simulink model "ISReferenceApplication"  (R2018a)
settings: Solver=FixedStepAuto  StartTime=0  StopTime=Tend  FixedStep=0.001  RelTol=5e-3
model workspace (MAT data in the model file):
  A_mu = 10
  B_reff = 8.386
  Cz = 7766.25
  DCT_Param : struct (value not decoded)
  D_reff = 0.25826
  Downshift_Speeds = [9.5625 12.9375 16.3125 19.6875 23.0625 26.4375 29.8125 33.1875 36.5625 39.9375 43.3125 46.6875 ... (28 elements, 4x7)]
  Pedal_Positions = [0.1 0.4 0.5 0.9]
  SUS : struct (value not decoded)
  Upshift_Speeds = [12.9375 16.3125 19.6875 33 26.4375 29.8125 33.1875 52.5 39.9375 43.3125 46.6875 77.25 ... (28 elements, 4x7)]
  VEH : struct (value not decoded)
  V_o = 16.7
  V_xlow = 1
  WH : struct (value not decoded)
  a = 1.4
  alpha_max = 1.5
  alpha_min = -1.5
  b = 1.8
  c_zo = 209651
  epsilon = 0.1
  h = 0.134
  path : struct (value not decoded)
  pio = 220000
  q_Fcx = 0
  q_Fz2 = 15.4
  q_Fzy = 0
  q_reo = 0.9974
  q_sx1 = -0.007764
  q_sx10 = 0.2824
  q_sx11 = 5.349
  q_sx12 = 0
  q_sx13 = 0
  q_sx14 = 0
  q_sx2 = 1.1915
  q_sx3 = 0.013948
  q_sx4 = 4.912
  q_sx5 = 1.02
  q_sx6 = 22.83
  q_sx7 = 0.7104
  q_sx8 = -0.023393
  q_sx9 = 0.6581
  q_sy1 = 0.00702
  q_sy2 = 0
  q_sy3 = 0.001515
  q_sy4 = 8.514e-05
  q_sy5 = 0
  q_sy6 = 0
  q_sy7 = 0.9008
  q_sy8 = -0.4089
  q_v1 = 0.0007742
  q_v2 = 0.04667
  r_Bx1 = 12.531
  r_Bx2 = 9.532
  r_Bx3 = 0
  r_By1 = 10.615
  r_By2 = 7.705
  r_By3 = 3.433e-06
  r_By4 = 0
  r_Cx1 = 1.019
  r_Cy1 = 1.0585
  r_Ex1 = -0.4487
  r_Ex2 = -0.4726
  r_Ey1 = 0.3132
  r_Ey2 = 7.63e-06
  r_Hx1 = 0.0002374
  r_Hy1 = 0.011646
  r_Hy2 = 7.63e-06
  r_Vy1 = 0.05654
  r_Vy2 = 7.63e-06
  r_Vy3 = 0
  r_Vy4 = 99.9
  r_Vy5 = 2
  r_Vy6 = 15.814
  r_o = 0.3135
  vehWidth = 2
  w = 1
undefined symbols (not defined in the file): Cok_1, Cok_2, Cok_3, Cok_4, Cok_5, Cok_6, Cok_7, Cok_8, Cok_9, Cout_1, Cout_2, Cout_3, Cout_4, Cout_5, Cout_6, Cout_7, Cout_8, Cout_9, Dout_1, Dout_2, Dout_3, Dout_4, Dout_5, Dout_6, Dout_7, Dout_8, Dout_9, F_1, F_2, F_3, F_4, F_5, F_6, F_7, F_8, F_9, Gd_1, Gd_2, Gd_3, Gd_4, Gd_5, Gd_6, Gd_7, Gd_8, Gd_9, Gok_1, Gok_2, Gok_3, Gok_4, Gok_5, Gok_6, Gok_7, Gok_8, Gok_9, Hd_1, Hd_2, Hd_3, Hd_4, Hd_5, Hd_6 ... (+64)
(part 2 of 3)

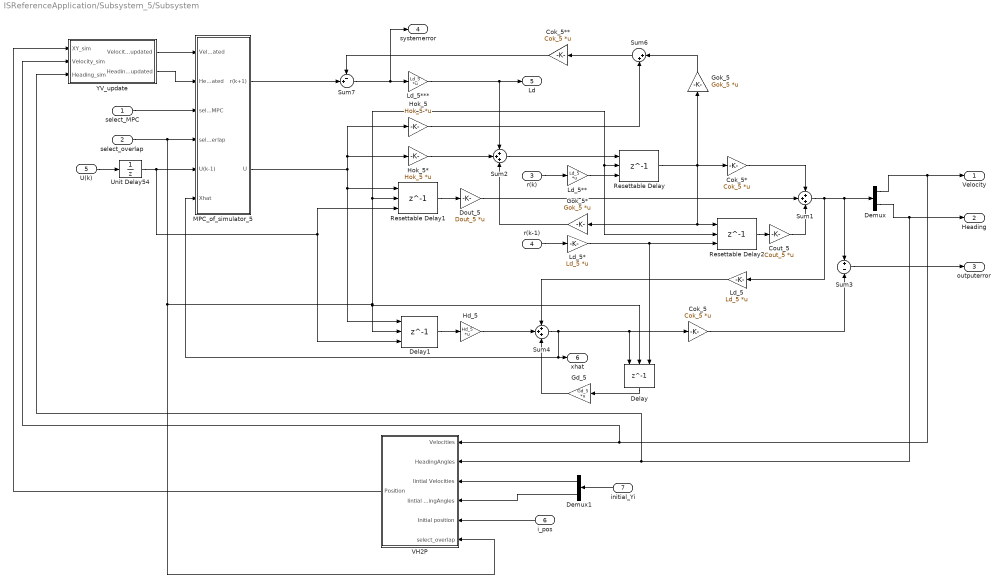
== system ISReferenceApplication/Subsystem_5/Subsystem ==
  select_MPC : Inport
  select_overlap : Inport  Port=2
  r(k) : Inport  Port=3
  r(k-1) : Inport  Port=4
  U(k) : Inport  Port=5
  i_pos : Inport  Port=6
  initial_Yi : Inport  Port=7
  Cok_5 : Gain  Gain=Cok_5  Multiplication=Matrix(K*u) (u vector)
  Cok_5* : Gain  Gain=Cok_5  Multiplication=Matrix(K*u) (u vector)
  Cok_5** : Gain  Gain=Cok_5  Multiplication=Matrix(K*u) (u vector)
  Cout_5 : Gain  Gain=Cout_5  Multiplication=Matrix(K*u) (u vector)
  Delay : Delay  DelayLength=1  InitialConditionSource=Input port  InitialCondition=0  ExternalReset=Rising  SampleTime=Ts
      settings: InputPortMap=u0,r5,p4
  Delay1 : Delay  DelayLength=1  InitialConditionSource=Input port  InitialCondition=0  ExternalReset=Rising  SampleTime=Ts
      settings: InputPortMap=u0,r5,p4
  Demux : Demux  Outputs=2
  Demux1 : Demux  Outputs=2
  Dout_5 : Gain  Gain=Dout_5  Multiplication=Matrix(K*u) (u vector)
  Gd_5 : Gain  Gain=Gd_5  Multiplication=Matrix(K*u) (u vector)
  Gok_5 : Gain  Gain=Gok_5  Multiplication=Matrix(K*u) (u vector)
  Gok_5* : Gain  Gain=Gok_5  Multiplication=Matrix(K*u) (u vector)
  Hd_5 : Gain  Gain=Hd_5  Multiplication=Matrix(K*u) (u vector)
  Hok_5 : Gain  Gain=Hok_5  Multiplication=Matrix(K*u) (u vector)
  Hok_5* : Gain  Gain=Hok_5  Multiplication=Matrix(K*u) (u vector)
  Ld_5 : Gain  Gain=Ld_5  Multiplication=Matrix(K*u) (u vector)
  Ld_5* : Gain  Gain=Ld_5  Multiplication=Matrix(K*u) (u vector)
  "Ld_5** " : Gain  Gain=Ld_5  Multiplication=Matrix(K*u) (u vector)
  Ld_5*** : Gain  Gain=Ld_5  Multiplication=Matrix(K*u) (u vector)
  MPC_of_simulator_5 : Subsystem
  Resettable Delay : Delay  DelayLength=1  InitialConditionSource=Input port  ExternalReset=Rising  SampleTime=Ts
      settings: InputPortMap=u0,r5,p4
  Resettable Delay1 : Delay  DelayLength=1  InitialConditionSource=Input port  ExternalReset=Rising  SampleTime=Ts
      settings: InputPortMap=u0,r5,p4
  Resettable Delay2 : Delay  DelayLength=1  InitialConditionSource=Input port  ExternalReset=Rising  SampleTime=Ts
      settings: InputPortMap=u0,r5,p4
  Sum1 : Sum  Inputs=+++
  Sum2 : Sum  Inputs=+++
  Sum3 : Sum  Inputs=+-
  Sum4 : Sum  Inputs=+++
  Sum6 : Sum  Inputs=|++
  Sum7 : Sum  Inputs=-+|
  Unit Delay54 : UnitDelay  SampleTime=Ts
  VH2P : Subsystem
  YV_update : Subsystem  TreatAsAtomicUnit=on
  Velocity : Outport
  Heading : Outport  Port=2
  outputerror : Outport  Port=3
  systemerror : Outport  Port=4
  Ld : Outport  Port=5
  xhat : Outport  Port=6
  wires:
  U(k)/1 -> Unit Delay54/1
  Cok_5*/1 -> Sum1/1
  Resettable Delay/1 -> Gok_5*/1, Resettable Delay2/1, Cok_5*/1, Gok_5/1
  Dout_5/1 -> Sum1/2
  Sum7/1 -> systemerror/1, Ld_5***/1
  r(k)/1 -> "Ld_5** "/1
  Gok_5*/1 -> Sum2/3
  Cout_5/1 -> Sum1/3
  Sum2/1 -> Resettable Delay/1
  "Ld_5** "/1 -> Resettable Delay/3
  Resettable Delay2/1 -> Cout_5/1
  r(k-1)/1 -> Ld_5*/1
  Hok_5/1 -> Sum6/2
  Gok_5/1 -> Sum6/1
  Resettable Delay1/1 -> Dout_5/1
  Sum6/1 -> Cok_5**/1
  Cok_5**/1 -> Sum7/1
  Hok_5*/1 -> Sum2/2
  Ld_5*/1 -> Resettable Delay2/3, Delay/3
  MPC_of_simulator_5/2(U) -> Hok_5/1, Hok_5*/1, Delay1/1, Resettable Delay1/1
  MPC_of_simulator_5/1(r(k+1)) -> Sum7/2
  Sum4/1 -> Cok_5/1, Delay/1, MPC_of_simulator_5/6(Xhat), xhat/1
  Gd_5/1 -> Sum4/3
  Delay/1 -> Gd_5/1
  Delay1/1 -> Hd_5/1
  Sum1/1 -> Ld_5/1, Sum3/1, Demux/1
  Cok_5/1 -> Sum3/2
  Hd_5/1 -> Sum4/2
  Ld_5***/1 -> Ld/1, Sum2/1
  Sum3/1 -> outputerror/1
  YV_update/1(Velocity_updated) -> MPC_of_simulator_5/1(Velocity_updated)
  YV_update/2(Heading_updated) -> MPC_of_simulator_5/2(Heading_updated)
  select_MPC/1 -> MPC_of_simulator_5/3(select_MPC)
  Demux/2 -> YV_update/3(Heading_sim), VH2P/2(HeadingAngles), Heading/1
  Demux/1 -> YV_update/2(Velocity_sim), VH2P/1(Velocities), Velocity/1
  VH2P/1(Position) -> YV_update/1(XY_sim)
  select_overlap/1 -> Resettable Delay2/2, Resettable Delay/2, Resettable Delay1/2, Delay/2, Delay1/2, VH2P/6(select_overlap), MPC_of_simulator_5/4(select_overlap)
  Unit Delay54/1 -> Resettable Delay1/3, Delay1/3, MPC_of_simulator_5/5(U(k-1))
  initial_Yi/1 -> Demux1/1
  Ld_5/1 -> Sum4/1
  i_pos/1 -> VH2P/5(Initial position)
  Demux1/1 -> VH2P/3(Iintial Velocities)
  Demux1/2 -> VH2P/4(Iintial HeadingAngles)

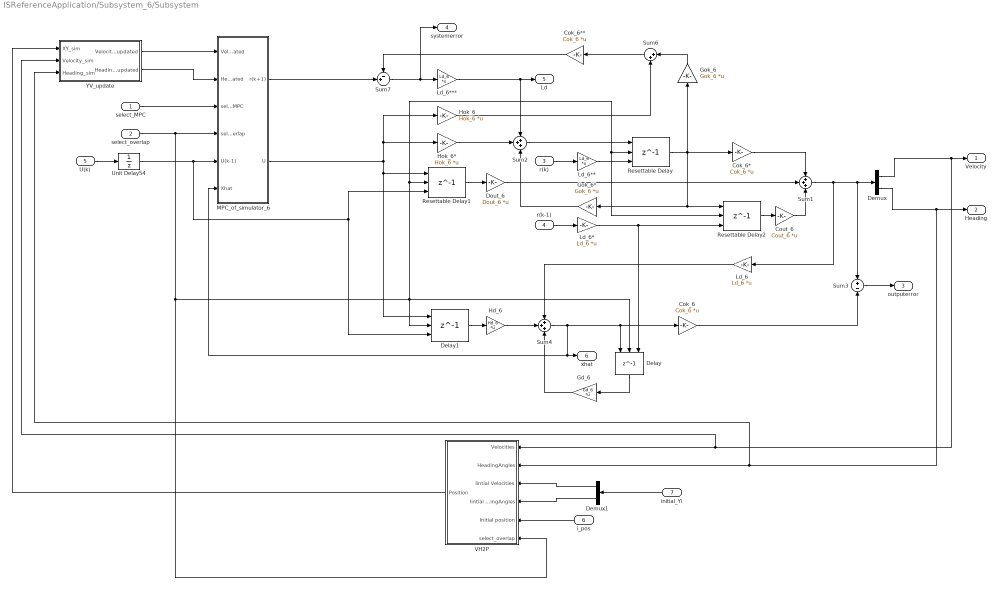
== system ISReferenceApplication/Subsystem_6/Subsystem ==
  select_MPC : Inport
  select_overlap : Inport  Port=2
  r(k) : Inport  Port=3
  r(k-1) : Inport  Port=4
  U(k) : Inport  Port=5
  i_pos : Inport  Port=6
  initial_Yi : Inport  Port=7
  Cok_6 : Gain  Gain=Cok_6  Multiplication=Matrix(K*u) (u vector)
  Cok_6* : Gain  Gain=Cok_6  Multiplication=Matrix(K*u) (u vector)
  Cok_6** : Gain  Gain=Cok_6  Multiplication=Matrix(K*u) (u vector)
  Cout_6 : Gain  Gain=Cout_6  Multiplication=Matrix(K*u) (u vector)
  Delay : Delay  DelayLength=1  InitialConditionSource=Input port  InitialCondition=0  ExternalReset=Rising  SampleTime=Ts
      settings: InputPortMap=u0,r5,p4
  Delay1 : Delay  DelayLength=1  InitialConditionSource=Input port  InitialCondition=0  ExternalReset=Rising  SampleTime=Ts
      settings: InputPortMap=u0,r5,p4
  Demux : Demux  Outputs=2
  Demux1 : Demux  Outputs=2
  Dout_6 : Gain  Gain=Dout_6  Multiplication=Matrix(K*u) (u vector)
  Gd_6 : Gain  Gain=Gd_6  Multiplication=Matrix(K*u) (u vector)
  Gok_6 : Gain  Gain=Gok_6  Multiplication=Matrix(K*u) (u vector)
  Gok_6* : Gain  Gain=Gok_6  Multiplication=Matrix(K*u) (u vector)
  Hd_6 : Gain  Gain=Hd_6  Multiplication=Matrix(K*u) (u vector)
  Hok_6 : Gain  Gain=Hok_6  Multiplication=Matrix(K*u) (u vector)
  Hok_6* : Gain  Gain=Hok_6  Multiplication=Matrix(K*u) (u vector)
  Ld_6 : Gain  Gain=Ld_6  Multiplication=Matrix(K*u) (u vector)
  Ld_6* : Gain  Gain=Ld_6  Multiplication=Matrix(K*u) (u vector)
  "Ld_6** " : Gain  Gain=Ld_6  Multiplication=Matrix(K*u) (u vector)
  Ld_6*** : Gain  Gain=Ld_6  Multiplication=Matrix(K*u) (u vector)
  MPC_of_simulator_6 : Subsystem
  Resettable Delay : Delay  DelayLength=1  InitialConditionSource=Input port  ExternalReset=Rising  SampleTime=Ts
      settings: InputPortMap=u0,r5,p4
  Resettable Delay1 : Delay  DelayLength=1  InitialConditionSource=Input port  ExternalReset=Rising  SampleTime=Ts
      settings: InputPortMap=u0,r5,p4
  Resettable Delay2 : Delay  DelayLength=1  InitialConditionSource=Input port  ExternalReset=Rising  SampleTime=Ts
      settings: InputPortMap=u0,r5,p4
  Sum1 : Sum  Inputs=+++
  Sum2 : Sum  Inputs=+++
  Sum3 : Sum  Inputs=+-
  Sum4 : Sum  Inputs=+++
  Sum6 : Sum  Inputs=|++
  Sum7 : Sum  Inputs=-+|
  Unit Delay54 : UnitDelay  SampleTime=Ts
  VH2P : Subsystem
  YV_update : Subsystem  TreatAsAtomicUnit=on
  Velocity : Outport
  Heading : Outport  Port=2
  outputerror : Outport  Port=3
  systemerror : Outport  Port=4
  Ld : Outport  Port=5
  xhat : Outport  Port=6
  wires:
  Sum2/1 -> Resettable Delay/1
  Sum6/1 -> Cok_6**/1
  Resettable Delay/1 -> Cok_6*/1, Resettable Delay2/1, Gok_6*/1, Gok_6/1
  Resettable Delay1/1 -> Dout_6/1
  Dout_6/1 -> Sum1/2
  Hok_6/1 -> Sum6/2
  MPC_of_simulator_6/2(U) -> Hok_6/1, Hok_6*/1, Delay1/1, Resettable Delay1/1
  r(k)/1 -> "Ld_6** "/1
  Sum1/1 -> Ld_6/1, Sum3/1, Demux/1
  Ld_6*/1 -> Resettable Delay2/3, Delay/3
  Hok_6*/1 -> Sum2/2
  Sum7/1 -> systemerror/1, Ld_6***/1
  Cok_6**/1 -> Sum7/1
  Cout_6/1 -> Sum1/3
  r(k-1)/1 -> Ld_6*/1
  Resettable Delay2/1 -> Cout_6/1
  "Ld_6** "/1 -> Resettable Delay/3
  Gok_6/1 -> Sum6/1
  Gok_6*/1 -> Sum2/3
  U(k)/1 -> Unit Delay54/1
  Ld_6***/1 -> Ld/1, Sum2/1
  Cok_6*/1 -> Sum1/1
  MPC_of_simulator_6/1(r(k+1)) -> Sum7/2
  Hd_6/1 -> Sum4/2
  Gd_6/1 -> Sum4/3
  Cok_6/1 -> Sum3/2
  Delay/1 -> Gd_6/1
  Delay1/1 -> Hd_6/1
  Sum4/1 -> Cok_6/1, Delay/1, MPC_of_simulator_6/6(Xhat), xhat/1
  Sum3/1 -> outputerror/1
  select_MPC/1 -> MPC_of_simulator_6/3(select_MPC)
  Demux/1 -> YV_update/2(Velocity_sim), VH2P/1(Velocities), Velocity/1
  VH2P/1(Position) -> YV_update/1(XY_sim)
  Demux/2 -> VH2P/2(HeadingAngles), YV_update/3(Heading_sim), Heading/1
  select_overlap/1 -> VH2P/6(select_overlap), Resettable Delay2/2, Resettable Delay/2, Resettable Delay1/2, Delay/2, Delay1/2, MPC_of_simulator_6/4(select_overlap)
  YV_update/1(Velocity_updated) -> MPC_of_simulator_6/1(Velocity_updated)
  YV_update/2(Heading_updated) -> MPC_of_simulator_6/2(Heading_updated)
  Unit Delay54/1 -> Resettable Delay1/3, Delay1/3, MPC_of_simulator_6/5(U(k-1))
  initial_Yi/1 -> Demux1/1
  Ld_6/1 -> Sum4/1
  i_pos/1 -> VH2P/5(Initial position)
  Demux1/1 -> VH2P/3(Iintial Velocities)
  Demux1/2 -> VH2P/4(Iintial HeadingAngles)

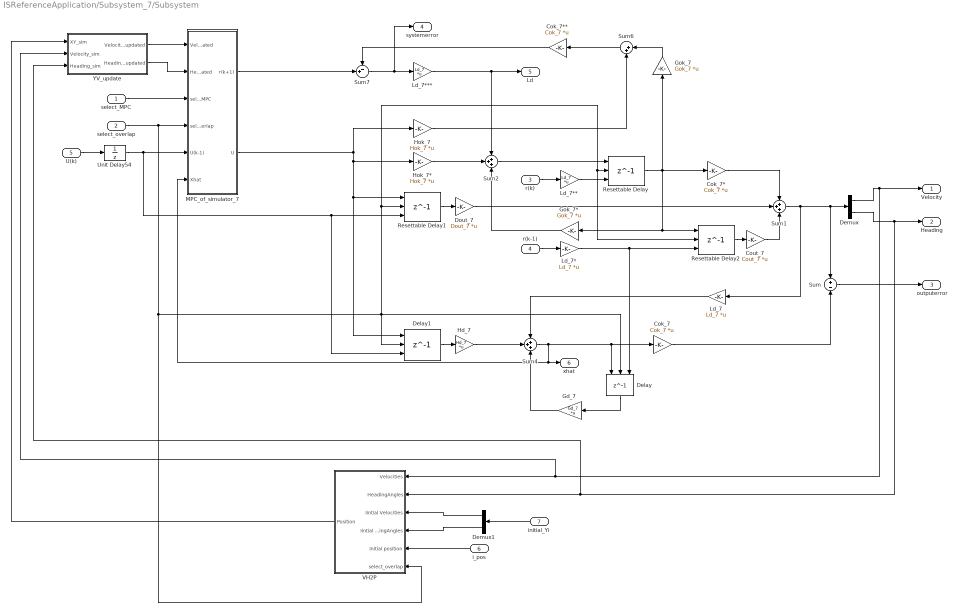
== system ISReferenceApplication/Subsystem_7/Subsystem ==
  select_MPC : Inport
  select_overlap : Inport  Port=2
  r(k) : Inport  Port=3
  r(k-1) : Inport  Port=4
  U(k) : Inport  Port=5
  i_pos : Inport  Port=6
  initial_Yi : Inport  Port=7
  Cok_7 : Gain  Gain=Cok_7  Multiplication=Matrix(K*u) (u vector)
  Cok_7* : Gain  Gain=Cok_7  Multiplication=Matrix(K*u) (u vector)
  Cok_7** : Gain  Gain=Cok_7  Multiplication=Matrix(K*u) (u vector)
  Cout_7 : Gain  Gain=Cout_7  Multiplication=Matrix(K*u) (u vector)
  Delay : Delay  DelayLength=1  InitialConditionSource=Input port  InitialCondition=0  ExternalReset=Rising  SampleTime=Ts
      settings: InputPortMap=u0,r5,p4
  Delay1 : Delay  DelayLength=1  InitialConditionSource=Input port  InitialCondition=0  ExternalReset=Rising  SampleTime=Ts
      settings: InputPortMap=u0,r5,p4
  Demux : Demux  Outputs=2
  Demux1 : Demux  Outputs=2
  Dout_7 : Gain  Gain=Dout_7  Multiplication=Matrix(K*u) (u vector)
  Gd_7 : Gain  Gain=Gd_7  Multiplication=Matrix(K*u) (u vector)
  Gok_7 : Gain  Gain=Gok_7  Multiplication=Matrix(K*u) (u vector)
  Gok_7* : Gain  Gain=Gok_7  Multiplication=Matrix(K*u) (u vector)
  Hd_7 : Gain  Gain=Hd_7  Multiplication=Matrix(K*u) (u vector)
  Hok_7 : Gain  Gain=Hok_7  Multiplication=Matrix(K*u) (u vector)
  Hok_7* : Gain  Gain=Hok_7  Multiplication=Matrix(K*u) (u vector)
  Ld_7 : Gain  Gain=Ld_7  Multiplication=Matrix(K*u) (u vector)
  Ld_7* : Gain  Gain=Ld_7  Multiplication=Matrix(K*u) (u vector)
  "Ld_7** " : Gain  Gain=Ld_7  Multiplication=Matrix(K*u) (u vector)
  Ld_7*** : Gain  Gain=Ld_7  Multiplication=Matrix(K*u) (u vector)
  MPC_of_simulator_7 : Subsystem
  Resettable Delay : Delay  DelayLength=1  InitialConditionSource=Input port  ExternalReset=Rising  SampleTime=Ts
      settings: InputPortMap=u0,r5,p4
  Resettable Delay1 : Delay  DelayLength=1  InitialConditionSource=Input port  ExternalReset=Rising  SampleTime=Ts
      settings: InputPortMap=u0,r5,p4
  Resettable Delay2 : Delay  DelayLength=1  InitialConditionSource=Input port  ExternalReset=Rising  SampleTime=Ts
      settings: InputPortMap=u0,r5,p4
  Sum : Sum  Inputs=+-
  Sum1 : Sum  Inputs=+++
  Sum2 : Sum  Inputs=+++
  Sum4 : Sum  Inputs=+++
  Sum6 : Sum  Inputs=|++
  Sum7 : Sum  Inputs=-+|
  Unit Delay54 : UnitDelay  SampleTime=Ts
  VH2P : Subsystem
  YV_update : Subsystem  TreatAsAtomicUnit=on
  Velocity : Outport
  Heading : Outport  Port=2
  outputerror : Outport  Port=3
  systemerror : Outport  Port=4
  Ld : Outport  Port=5
  xhat : Outport  Port=6
  wires:
  "Ld_7** "/1 -> Resettable Delay/3
  Dout_7/1 -> Sum1/2
  Resettable Delay1/1 -> Dout_7/1
  Cout_7/1 -> Sum1/3
  U(k)/1 -> Unit Delay54/1
  Ld_7***/1 -> Ld/1, Sum2/1
  Gok_7*/1 -> Sum2/3
  Resettable Delay/1 -> Resettable Delay2/1, Gok_7*/1, Cok_7*/1, Gok_7/1
  Cok_7**/1 -> Sum7/1
  r(k-1)/1 -> Ld_7*/1
  Sum7/1 -> Ld_7***/1, systemerror/1
  Sum1/1 -> Ld_7/1, Sum/1, Demux/1
  Resettable Delay2/1 -> Cout_7/1
  Sum6/1 -> Cok_7**/1
  Cok_7*/1 -> Sum1/1
  Hok_7/1 -> Sum6/2
  Gok_7/1 -> Sum6/1
  Ld_7*/1 -> Resettable Delay2/3, Delay/3
  MPC_of_simulator_7/1(r(k+1)) -> Sum7/2
  r(k)/1 -> "Ld_7** "/1
  Hok_7*/1 -> Sum2/2
  MPC_of_simulator_7/2(U) -> Hok_7/1, Delay1/1, Resettable Delay1/1, Hok_7*/1
  Sum2/1 -> Resettable Delay/1
  Delay/1 -> Gd_7/1
  Sum4/1 -> Cok_7/1, Delay/1, MPC_of_simulator_7/6(Xhat), xhat/1
  Hd_7/1 -> Sum4/2
  Delay1/1 -> Hd_7/1
  Cok_7/1 -> Sum/2
  Gd_7/1 -> Sum4/3
  Sum/1 -> outputerror/1
  Demux/1 -> YV_update/2(Velocity_sim), VH2P/1(Velocities), Velocity/1
  VH2P/1(Position) -> YV_update/1(XY_sim)
  select_overlap/1 -> VH2P/6(select_overlap), Delay1/2, Resettable Delay2/2, Resettable Delay/2, Resettable Delay1/2, Delay/2, MPC_of_simulator_7/4(select_overlap)
  Demux/2 -> YV_update/3(Heading_sim), VH2P/2(HeadingAngles), Heading/1
  YV_update/1(Velocity_updated) -> MPC_of_simulator_7/1(Velocity_updated)
  YV_update/2(Heading_updated) -> MPC_of_simulator_7/2(Heading_updated)
  select_MPC/1 -> MPC_of_simulator_7/3(select_MPC)
  Unit Delay54/1 -> MPC_of_simulator_7/5(U(k-1)), Resettable Delay1/3, Delay1/3
  Ld_7/1 -> Sum4/1
  initial_Yi/1 -> Demux1/1
  i_pos/1 -> VH2P/5(Initial position)
  Demux1/1 -> VH2P/3(Iintial Velocities)
  Demux1/2 -> VH2P/4(Iintial HeadingAngles)

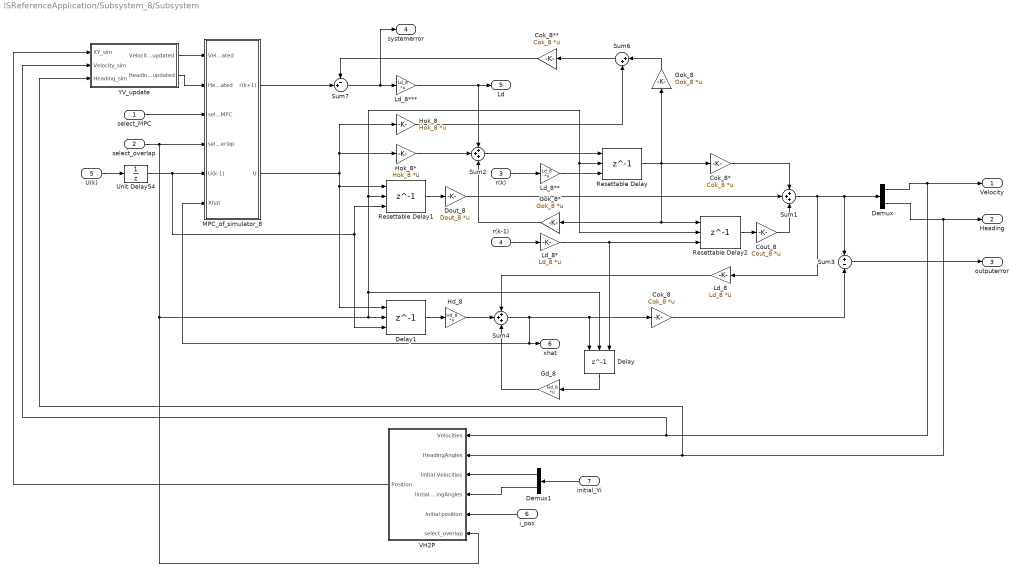
== system ISReferenceApplication/Subsystem_8/Subsystem ==
  select_MPC : Inport
  select_overlap : Inport  Port=2
  r(k) : Inport  Port=3
  r(k-1) : Inport  Port=4
  U(k) : Inport  Port=5
  i_pos : Inport  Port=6
  initial_Yi : Inport  Port=7
  Cok_8 : Gain  Gain=Cok_8  Multiplication=Matrix(K*u) (u vector)
  Cok_8* : Gain  Gain=Cok_8  Multiplication=Matrix(K*u) (u vector)
  Cok_8** : Gain  Gain=Cok_8  Multiplication=Matrix(K*u) (u vector)
  Cout_8 : Gain  Gain=Cout_8  Multiplication=Matrix(K*u) (u vector)
  Delay : Delay  DelayLength=1  InitialConditionSource=Input port  InitialCondition=0  ExternalReset=Rising  SampleTime=Ts
      settings: InputPortMap=u0,r5,p4
  Delay1 : Delay  DelayLength=1  InitialConditionSource=Input port  InitialCondition=0  ExternalReset=Rising  SampleTime=Ts
      settings: InputPortMap=u0,r5,p4
  Demux : Demux  Outputs=2
  Demux1 : Demux  Outputs=2
  Dout_8 : Gain  Gain=Dout_8  Multiplication=Matrix(K*u) (u vector)
  Gd_8 : Gain  Gain=Gd_8  Multiplication=Matrix(K*u) (u vector)
  Gok_8 : Gain  Gain=Gok_8  Multiplication=Matrix(K*u) (u vector)
  Gok_8* : Gain  Gain=Gok_8  Multiplication=Matrix(K*u) (u vector)
  Hd_8 : Gain  Gain=Hd_8  Multiplication=Matrix(K*u) (u vector)
  Hok_8 : Gain  Gain=Hok_8  Multiplication=Matrix(K*u) (u vector)
  Hok_8* : Gain  Gain=Hok_8  Multiplication=Matrix(K*u) (u vector)
  Ld_8 : Gain  Gain=Ld_8  Multiplication=Matrix(K*u) (u vector)
  Ld_8* : Gain  Gain=Ld_8  Multiplication=Matrix(K*u) (u vector)
  "Ld_8** " : Gain  Gain=Ld_8  Multiplication=Matrix(K*u) (u vector)
  Ld_8*** : Gain  Gain=Ld_8  Multiplication=Matrix(K*u) (u vector)
  MPC_of_simulator_8 : Subsystem
  Resettable Delay : Delay  DelayLength=1  InitialConditionSource=Input port  ExternalReset=Rising  SampleTime=Ts
      settings: InputPortMap=u0,r5,p4
  Resettable Delay1 : Delay  DelayLength=1  InitialConditionSource=Input port  ExternalReset=Rising  SampleTime=Ts
      settings: InputPortMap=u0,r5,p4
  Resettable Delay2 : Delay  DelayLength=1  InitialConditionSource=Input port  ExternalReset=Rising  SampleTime=Ts
      settings: InputPortMap=u0,r5,p4
  Sum1 : Sum  Inputs=+++
  Sum2 : Sum  Inputs=+++
  Sum3 : Sum  Inputs=+-
  Sum4 : Sum  Inputs=+++
  Sum6 : Sum  Inputs=|++
  Sum7 : Sum  Inputs=-+|
  Unit Delay54 : UnitDelay  SampleTime=Ts
  VH2P : Subsystem
  YV_update : Subsystem  TreatAsAtomicUnit=on
  Velocity : Outport
  Heading : Outport  Port=2
  outputerror : Outport  Port=3
  systemerror : Outport  Port=4
  Ld : Outport  Port=5
  xhat : Outport  Port=6
  wires:
  Hok_8/1 -> Sum6/2
  Resettable Delay/1 -> Cok_8*/1, Resettable Delay2/1, Gok_8*/1, Gok_8/1
  Sum7/1 -> systemerror/1, Ld_8***/1
  Cok_8**/1 -> Sum7/1
  Gok_8*/1 -> Sum2/3
  Cok_8*/1 -> Sum1/1
  r(k)/1 -> "Ld_8** "/1
  Resettable Delay2/1 -> Cout_8/1
  "Ld_8** "/1 -> Resettable Delay/3
  Ld_8***/1 -> Ld/1, Sum2/1
  Dout_8/1 -> Sum1/2
  Resettable Delay1/1 -> Dout_8/1
  Gok_8/1 -> Sum6/1
  Ld_8*/1 -> Resettable Delay2/3, Delay/3
  Sum6/1 -> Cok_8**/1
  Sum1/1 -> Ld_8/1, Sum3/1, Demux/1
  r(k-1)/1 -> Ld_8*/1
  Sum2/1 -> Resettable Delay/1
  Cout_8/1 -> Sum1/3
  Hok_8*/1 -> Sum2/2
  MPC_of_simulator_8/1(r(k+1)) -> Sum7/2
  MPC_of_simulator_8/2(U) -> Hok_8/1, Hok_8*/1, Delay1/1, Resettable Delay1/1
  Hd_8/1 -> Sum4/2
  Gd_8/1 -> Sum4/3
  Delay/1 -> Gd_8/1
  Delay1/1 -> Hd_8/1
  Cok_8/1 -> Sum3/2
  Sum4/1 -> Cok_8/1, Delay/1, xhat/1, MPC_of_simulator_8/6(Xhat)
  U(k)/1 -> Unit Delay54/1
  Sum3/1 -> outputerror/1
  YV_update/1(Velocity_updated) -> MPC_of_simulator_8/1(Velocity_updated)
  VH2P/1(Position) -> YV_update/1(XY_sim)
  Demux/1 -> YV_update/2(Velocity_sim), VH2P/1(Velocities), Velocity/1
  Demux/2 -> YV_update/3(Heading_sim), VH2P/2(HeadingAngles), Heading/1
  select_overlap/1 -> MPC_of_simulator_8/4(select_overlap), VH2P/6(select_overlap), Resettable Delay2/2, Resettable Delay/2, Resettable Delay1/2, Delay/2, Delay1/2
  YV_update/2(Heading_updated) -> MPC_of_simulator_8/2(Heading_updated)
  select_MPC/1 -> MPC_of_simulator_8/3(select_MPC)
  Unit Delay54/1 -> Delay1/3, Resettable Delay1/3, MPC_of_simulator_8/5(U(k-1))
  initial_Yi/1 -> Demux1/1
  Ld_8/1 -> Sum4/1
  i_pos/1 -> VH2P/5(Initial position)
  Demux1/1 -> VH2P/3(Iintial Velocities)
  Demux1/2 -> VH2P/4(Iintial HeadingAngles)

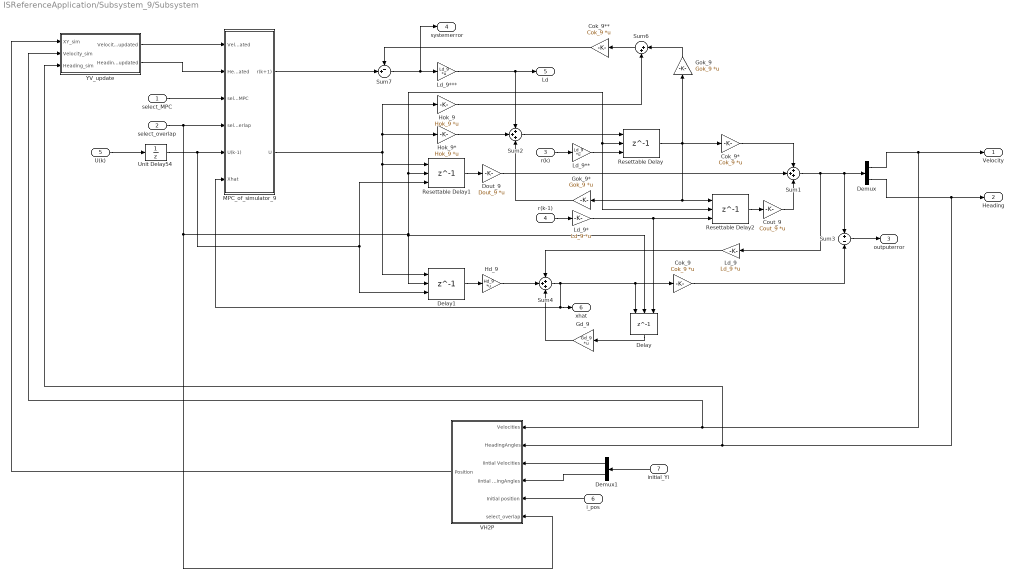
== system ISReferenceApplication/Subsystem_9/Subsystem ==
  select_MPC : Inport
  select_overlap : Inport  Port=2
  r(k) : Inport  Port=3
  r(k-1) : Inport  Port=4
  U(k) : Inport  Port=5
  i_pos : Inport  Port=6
  initial_Yi : Inport  Port=7
  Cok_9 : Gain  Gain=Cok_9  Multiplication=Matrix(K*u) (u vector)
  Cok_9* : Gain  Gain=Cok_9  Multiplication=Matrix(K*u) (u vector)
  Cok_9** : Gain  Gain=Cok_9  Multiplication=Matrix(K*u) (u vector)
  Cout_9 : Gain  Gain=Cout_9  Multiplication=Matrix(K*u) (u vector)
  Delay : Delay  DelayLength=1  InitialConditionSource=Input port  InitialCondition=0  ExternalReset=Rising  SampleTime=Ts
      settings: InputPortMap=u0,r5,p4
  Delay1 : Delay  DelayLength=1  InitialConditionSource=Input port  InitialCondition=0  ExternalReset=Rising  SampleTime=Ts
      settings: InputPortMap=u0,r5,p4
  Demux : Demux  Outputs=2
  Demux1 : Demux  Outputs=2
  Dout_9 : Gain  Gain=Dout_9  Multiplication=Matrix(K*u) (u vector)
  Gd_9 : Gain  Gain=Gd_9  Multiplication=Matrix(K*u) (u vector)
  Gok_9 : Gain  Gain=Gok_9  Multiplication=Matrix(K*u) (u vector)
  Gok_9* : Gain  Gain=Gok_9  Multiplication=Matrix(K*u) (u vector)
  Hd_9 : Gain  Gain=Hd_9  Multiplication=Matrix(K*u) (u vector)
  Hok_9 : Gain  Gain=Hok_9  Multiplication=Matrix(K*u) (u vector)
  Hok_9* : Gain  Gain=Hok_9  Multiplication=Matrix(K*u) (u vector)
  Ld_9 : Gain  Gain=Ld_9  Multiplication=Matrix(K*u) (u vector)
  Ld_9* : Gain  Gain=Ld_9  Multiplication=Matrix(K*u) (u vector)
  "Ld_9** " : Gain  Gain=Ld_9  Multiplication=Matrix(K*u) (u vector)
  Ld_9*** : Gain  Gain=Ld_9  Multiplication=Matrix(K*u) (u vector)
  MPC_of_simulator_9 : Subsystem
  Resettable Delay : Delay  DelayLength=1  InitialConditionSource=Input port  ExternalReset=Rising  SampleTime=Ts
      settings: InputPortMap=u0,r5,p4
  Resettable Delay1 : Delay  DelayLength=1  InitialConditionSource=Input port  ExternalReset=Rising  SampleTime=Ts
      settings: InputPortMap=u0,r5,p4
  Resettable Delay2 : Delay  DelayLength=1  InitialConditionSource=Input port  ExternalReset=Rising  SampleTime=Ts
      settings: InputPortMap=u0,r5,p4
  Sum1 : Sum  Inputs=+++
  Sum2 : Sum  Inputs=+++
  Sum3 : Sum  Inputs=+-
  Sum4 : Sum  Inputs=+++
  Sum6 : Sum  Inputs=|++
  Sum7 : Sum  Inputs=-+|
  Unit Delay54 : UnitDelay  SampleTime=Ts
  VH2P : Subsystem
  YV_update : Subsystem  TreatAsAtomicUnit=on
  Velocity : Outport
  Heading : Outport  Port=2
  outputerror : Outport  Port=3
  systemerror : Outport  Port=4
  Ld : Outport  Port=5
  xhat : Outport  Port=6
  wires:
  select_overlap/1 -> MPC_of_simulator_9/4(select_overlap), VH2P/6(select_overlap), Resettable Delay2/2, Resettable Delay/2, Resettable Delay1/2, Delay/2, Delay1/2
  Hok_9/1 -> Sum6/2
  Resettable Delay/1 -> Cok_9*/1, Resettable Delay2/1, Gok_9*/1, Gok_9/1
  Sum7/1 -> systemerror/1, Ld_9***/1
  Cok_9**/1 -> Sum7/1
  Gok_9*/1 -> Sum2/3
  Cok_9*/1 -> Sum1/1
  r(k)/1 -> "Ld_9** "/1
  Resettable Delay2/1 -> Cout_9/1
  "Ld_9** "/1 -> Resettable Delay/3
  Ld_9***/1 -> Ld/1, Sum2/1
  Dout_9/1 -> Sum1/2
  Resettable Delay1/1 -> Dout_9/1
  Gok_9/1 -> Sum6/1
  Ld_9*/1 -> Delay/3, Resettable Delay2/3
  Sum6/1 -> Cok_9**/1
  Sum1/1 -> Sum3/1, Demux/1, Ld_9/1
  r(k-1)/1 -> Ld_9*/1
  Sum2/1 -> Resettable Delay/1
  Cout_9/1 -> Sum1/3
  Demux/2 -> YV_update/3(Heading_sim), VH2P/2(HeadingAngles), Heading/1
  Hok_9*/1 -> Sum2/2
  Demux/1 -> YV_update/2(Velocity_sim), VH2P/1(Velocities), Velocity/1
  MPC_of_simulator_9/2(U) -> Hok_9/1, Hok_9*/1, Resettable Delay1/1, Delay1/1
  Hd_9/1 -> Sum4/2
  Gd_9/1 -> Sum4/3
  Ld_9/1 -> Sum4/1
  Delay/1 -> Gd_9/1
  Delay1/1 -> Hd_9/1
  Cok_9/1 -> Sum3/2
  Sum4/1 -> Cok_9/1, Delay/1, xhat/1, MPC_of_simulator_9/6(Xhat)
  Unit Delay54/1 -> MPC_of_simulator_9/5(U(k-1)), Resettable Delay1/3, Delay1/3
  Sum3/1 -> outputerror/1
  select_MPC/1 -> MPC_of_simulator_9/3(select_MPC)
  YV_update/1(Velocity_updated) -> MPC_of_simulator_9/1(Velocity_updated)
  YV_update/2(Heading_updated) -> MPC_of_simulator_9/2(Heading_updated)
  MPC_of_simulator_9/1(r(k+1)) -> Sum7/2
  U(k)/1 -> Unit Delay54/1
  VH2P/1(Position) -> YV_update/1(XY_sim)
  initial_Yi/1 -> Demux1/1
  Demux1/1 -> VH2P/3(Iintial Velocities)
  Demux1/2 -> VH2P/4(Iintial HeadingAngles)
  i_pos/1 -> VH2P/5(Initial position)

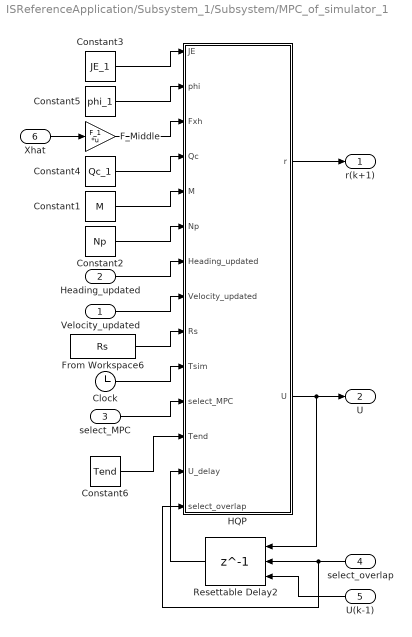
== system ISReferenceApplication/Subsystem_1/Subsystem/MPC_of_simulator_1 ==
  Velocity_updated : Inport  SampleTime=Ts  LockScale=on
  Heading_updated : Inport  Port=2  SampleTime=Ts  LockScale=on
  select_MPC : Inport  Port=3  SampleTime=Ts  LockScale=on
  select_overlap : Inport  Port=4  SampleTime=Ts  LockScale=on
  U(k-1) : Inport  Port=5  SampleTime=Ts  LockScale=on
  Xhat : Inport  Port=6
  Clock : Clock
  Constant1 : Constant  Value=M  VectorParams1D=off  SampleTime=-1
  Constant2 : Constant  Value=Np  SampleTime=-1
  Constant3 : Constant  Value=JE_1  VectorParams1D=off  SampleTime=-1
  Constant4 : Constant  Value=Qc_1  VectorParams1D=off  SampleTime=-1
  Constant5 : Constant  Value=phi_1  VectorParams1D=off  SampleTime=-1
  Constant6 : Constant  Value=Tend  SampleTime=-1
  F_Middle : Gain  Gain=F_1  Multiplication=Matrix(K*u) (u vector)
  From Workspace6 : FromWorkspace  VariableName=Rs  SampleTime=Ts
  HQP : MATLAB Function  TreatAsAtomicUnit=on  SystemSampleTime=Ts
  Resettable Delay2 : Delay  DelayLength=1  InitialConditionSource=Input port  ExternalReset=Rising  SampleTime=Ts
      settings: InputPortMap=u0,r5,p4
  r(k+1) : Outport
  U : Outport  Port=2
  wires:
  HQP/2(U) -> Resettable Delay2/1, U/1
  Xhat/1 -> F_Middle/1
  Constant4/1 -> HQP/4(Qc)
  Constant5/1 -> HQP/2(phi)
  Constant3/1 -> HQP/1(JE)
  Constant2/1 -> HQP/6(Np)
  Constant1/1 -> HQP/5(M)
  Clock/1 -> HQP/10(Tsim)
  F_Middle/1 -> HQP/3(Fxh)
  From Workspace6/1 -> HQP/9(Rs)
  Heading_updated/1 -> HQP/7(Heading_updated)
  Velocity_updated/1 -> HQP/8(Velocity_updated)
  HQP/1(r) -> r(k+1)/1
  select_MPC/1 -> HQP/11(select_MPC)
  Resettable Delay2/1 -> HQP/13(U_delay)
  select_overlap/1 -> HQP/14(select_overlap), Resettable Delay2/2
  U(k-1)/1 -> Resettable Delay2/3
  Constant6/1 -> HQP/12(Tend)

== system ISReferenceApplication/Subsystem_1/Subsystem/VH2P ==
  Velocities : Inport
  HeadingAngles : Inport  Port=2
  Iintial Velocities : Inport  Port=3
  Iintial HeadingAngles : Inport  Port=4
  Initial position : Inport  Port=5
  select_overlap : Inport  Port=6
  Delay1 : Delay  DelayLength=1  InitialConditionSource=Input port  InitialCondition=0  ExternalReset=Rising  SampleTime=Ts
      settings: InputPortMap=u0,r5,p4
  Delay2 : Delay  DelayLength=1  InitialConditionSource=Input port  InitialCondition=0  ExternalReset=Rising  SampleTime=Ts
      settings: InputPortMap=u0,r5,p4
  Delay3 : Delay  DelayLength=1  InitialConditionSource=Input port  InitialCondition=0  ExternalReset=Rising  SampleTime=Ts
      settings: InputPortMap=u0,r5,p4
  From Workspace : FromWorkspace  VariableName=T_sim  SampleTime=Ts
  Unit Delay3 : UnitDelay  SampleTime=Ts
  YV2P : MATLAB Function  TreatAsAtomicUnit=on  SystemSampleTime=Ts
  Position : Outport
  wires:
  Velocities/1 -> YV2P/1(Velocity), Delay1/1
  HeadingAngles/1 -> Delay3/1, YV2P/3(Yaw)
  Delay2/1 -> YV2P/7(Lastpostion)
  Initial position/1 -> Delay2/3
  Iintial Velocities/1 -> Delay1/3
  Iintial HeadingAngles/1 -> Delay3/3
  From Workspace/1 -> YV2P/5(Tsim), Unit Delay3/1
  Delay1/1 -> YV2P/2(LastVelocity)
  Delay3/1 -> YV2P/4(LastYaw)
  Unit Delay3/1 -> YV2P/6(LastTsim)
  YV2P/1(Position) -> Delay2/1, Position/1
  select_overlap/1 -> Delay2/2, Delay1/2, Delay3/2

== system ISReferenceApplication/Subsystem_1/Subsystem/YV_update ==
  XY_sim : Inport
  Velocity_sim : Inport  Port=2
  Heading_sim : Inport  Port=3
  Constant : Constant  Value=Ts  SampleTime=Ts
  From Workspace1 : FromWorkspace  VariableName=T_sim  SampleTime=Ts
  From Workspace3 : FromWorkspace  VariableName=XY_Ref_Upd  SampleTime=Ts
  YV_update : MATLAB Function  TreatAsAtomicUnit=on  SystemSampleTime=Ts
  Velocity_updated : Outport
  Heading_updated : Outport  Port=2
  wires:
  YV_update/1(Velocity_updated) -> Velocity_updated/1
  From Workspace3/1 -> YV_update/1(XYplot_ref)
  YV_update/2(Heading_updated) -> Heading_updated/1
  From Workspace1/1 -> YV_update/6(Tsim)
  XY_sim/1 -> YV_update/2(XYplot_sim)
  Velocity_sim/1 -> YV_update/3(Velocity_sim)
  Heading_sim/1 -> YV_update/4(Heading_sim)
  Constant/1 -> YV_update/5(Ts)

== system ISReferenceApplication/Subsystem_2/Subsystem/MPC_of_simulator_2 ==
  Velocity_updated : Inport  SampleTime=Ts  LockScale=on
  Heading_updated : Inport  Port=2  SampleTime=Ts  LockScale=on
  select_MPC : Inport  Port=3  SampleTime=Ts  LockScale=on
  select_overlap : Inport  Port=4  SampleTime=Ts  LockScale=on
  U(k-1) : Inport  Port=5  SampleTime=Ts  LockScale=on
  Xhat : Inport  Port=6
  Clock : Clock
  Constant1 : Constant  Value=M  VectorParams1D=off  SampleTime=-1
  Constant2 : Constant  Value=Np  SampleTime=-1
  Constant3 : Constant  Value=JE_2  VectorParams1D=off  SampleTime=-1
  Constant4 : Constant  Value=Qc_2  VectorParams1D=off  SampleTime=-1
  Constant5 : Constant  Value=phi_2  VectorParams1D=off  SampleTime=-1
  Constant6 : Constant  Value=Tend  SampleTime=-1
  F_Middle : Gain  Gain=F_2  Multiplication=Matrix(K*u) (u vector)
  From Workspace6 : FromWorkspace  VariableName=Rs  SampleTime=Ts
  HQP : MATLAB Function  TreatAsAtomicUnit=on  SystemSampleTime=Ts
  Resettable Delay2 : Delay  DelayLength=1  InitialConditionSource=Input port  ExternalReset=Rising  SampleTime=Ts
      settings: InputPortMap=u0,r5,p4
  r(k+1) : Outport
  U : Outport  Port=2
  wires:
  HQP/2(U) -> Resettable Delay2/1, U/1
  Xhat/1 -> F_Middle/1
  Constant4/1 -> HQP/4(Qc)
  Constant5/1 -> HQP/2(phi)
  Constant3/1 -> HQP/1(JE)
  Constant2/1 -> HQP/6(Np)
  Constant1/1 -> HQP/5(M)
  Clock/1 -> HQP/10(Tsim)
  F_Middle/1 -> HQP/3(Fxh)
  From Workspace6/1 -> HQP/9(Rs)
  Heading_updated/1 -> HQP/7(Heading_updated)
  Velocity_updated/1 -> HQP/8(Velocity_updated)
  HQP/1(r) -> r(k+1)/1
  select_MPC/1 -> HQP/11(select_MPC)
  Resettable Delay2/1 -> HQP/13(U_delay)
  select_overlap/1 -> Resettable Delay2/2
  U(k-1)/1 -> Resettable Delay2/3
  Constant6/1 -> HQP/12(Tend)

== system ISReferenceApplication/Subsystem_2/Subsystem/VH2P ==
  Velocities : Inport
  HeadingAngles : Inport  Port=2
  Iintial Velocities : Inport  Port=3
  Iintial HeadingAngles : Inport  Port=4
  Initial position : Inport  Port=5
  select_overlap : Inport  Port=6
  Delay1 : Delay  DelayLength=1  InitialConditionSource=Input port  InitialCondition=0  ExternalReset=Rising  SampleTime=Ts
      settings: InputPortMap=u0,r5,p4
  Delay2 : Delay  DelayLength=1  InitialConditionSource=Input port  InitialCondition=0  ExternalReset=Rising  SampleTime=Ts
      settings: InputPortMap=u0,r5,p4
  Delay3 : Delay  DelayLength=1  InitialConditionSource=Input port  InitialCondition=0  ExternalReset=Rising  SampleTime=Ts
      settings: InputPortMap=u0,r5,p4
  From Workspace : FromWorkspace  VariableName=T_sim  SampleTime=Ts
  Unit Delay3 : UnitDelay  SampleTime=Ts
  YV2P : MATLAB Function  TreatAsAtomicUnit=on  SystemSampleTime=Ts
  Position : Outport
  wires:
  Velocities/1 -> YV2P/1(Velocity), Delay1/1
  HeadingAngles/1 -> Delay3/1, YV2P/3(Yaw)
  Delay2/1 -> YV2P/7(Lastpostion)
  Initial position/1 -> Delay2/3
  Iintial Velocities/1 -> Delay1/3
  Iintial HeadingAngles/1 -> Delay3/3
  From Workspace/1 -> YV2P/5(Tsim), Unit Delay3/1
  Delay1/1 -> YV2P/2(LastVelocity)
  Delay3/1 -> YV2P/4(LastYaw)
  Unit Delay3/1 -> YV2P/6(LastTsim)
  YV2P/1(Position) -> Delay2/1, Position/1
  select_overlap/1 -> Delay2/2, Delay1/2, Delay3/2

== system ISReferenceApplication/Subsystem_2/Subsystem/YV_update ==
  XY_sim : Inport
  Velocity_sim : Inport  Port=2
  Heading_sim : Inport  Port=3
  Constant : Constant  Value=Ts  SampleTime=Ts
  From Workspace1 : FromWorkspace  VariableName=T_sim  SampleTime=Ts
  From Workspace3 : FromWorkspace  VariableName=XY_Ref_Upd  SampleTime=Ts
  YV_update : MATLAB Function  TreatAsAtomicUnit=on  SystemSampleTime=Ts
  Velocity_updated : Outport
  Heading_updated : Outport  Port=2
  wires:
  YV_update/1(Velocity_updated) -> Velocity_updated/1
  From Workspace3/1 -> YV_update/1(XYplot_ref)
  YV_update/2(Heading_updated) -> Heading_updated/1
  From Workspace1/1 -> YV_update/6(Tsim)
  XY_sim/1 -> YV_update/2(XYplot_sim)
  Velocity_sim/1 -> YV_update/3(Velocity_sim)
  Heading_sim/1 -> YV_update/4(Heading_sim)
  Constant/1 -> YV_update/5(Ts)

== system ISReferenceApplication/Subsystem_3/Subsystem/MPC_of_simulator_3 ==
  Velocity_updated : Inport  SampleTime=Ts  LockScale=on
  Heading_updated : Inport  Port=2  SampleTime=Ts  LockScale=on
  select_MPC : Inport  Port=3  SampleTime=Ts  LockScale=on
  select_overlap : Inport  Port=4  SampleTime=Ts  LockScale=on
  U(k-1) : Inport  Port=5  SampleTime=Ts  LockScale=on
  Xhat : Inport  Port=6
  Clock : Clock
  Constant1 : Constant  Value=M  VectorParams1D=off  SampleTime=-1
  Constant2 : Constant  Value=Np  SampleTime=-1
  Constant3 : Constant  Value=JE_3  VectorParams1D=off  SampleTime=-1
  Constant4 : Constant  Value=Qc_3  VectorParams1D=off  SampleTime=-1
  Constant5 : Constant  Value=phi_3  VectorParams1D=off  SampleTime=-1
  Constant6 : Constant  Value=Tend  SampleTime=-1
  F_Middle : Gain  Gain=F_3  Multiplication=Matrix(K*u) (u vector)
  From Workspace6 : FromWorkspace  VariableName=Rs  SampleTime=Ts
  HQP : MATLAB Function  TreatAsAtomicUnit=on  SystemSampleTime=Ts
  Resettable Delay2 : Delay  DelayLength=1  InitialConditionSource=Input port  ExternalReset=Rising  SampleTime=Ts
      settings: InputPortMap=u0,r5,p4
  r(k+1) : Outport
  U : Outport  Port=2
  wires:
  HQP/2(U) -> Resettable Delay2/1, U/1
  Xhat/1 -> F_Middle/1
  Constant4/1 -> HQP/4(Qc)
  Constant5/1 -> HQP/2(phi)
  Constant3/1 -> HQP/1(JE)
  Constant2/1 -> HQP/6(Np)
  Constant1/1 -> HQP/5(M)
  Clock/1 -> HQP/10(Tsim)
  F_Middle/1 -> HQP/3(Fxh)
  From Workspace6/1 -> HQP/9(Rs)
  Heading_updated/1 -> HQP/7(Heading_updated)
  Velocity_updated/1 -> HQP/8(Velocity_updated)
  HQP/1(r) -> r(k+1)/1
  select_MPC/1 -> HQP/11(select_MPC)
  Resettable Delay2/1 -> HQP/13(U_delay)
  select_overlap/1 -> HQP/14(select_overlap), Resettable Delay2/2
  U(k-1)/1 -> Resettable Delay2/3
  Constant6/1 -> HQP/12(Tend)

== system ISReferenceApplication/Subsystem_3/Subsystem/VH2P ==
  Velocities : Inport
  HeadingAngles : Inport  Port=2
  Iintial Velocities : Inport  Port=3
  Iintial HeadingAngles : Inport  Port=4
  Initial position : Inport  Port=5
  select_overlap : Inport  Port=6
  Delay1 : Delay  DelayLength=1  InitialConditionSource=Input port  InitialCondition=0  ExternalReset=Rising  SampleTime=Ts
      settings: InputPortMap=u0,r5,p4
  Delay2 : Delay  DelayLength=1  InitialConditionSource=Input port  InitialCondition=0  ExternalReset=Rising  SampleTime=Ts
      settings: InputPortMap=u0,r5,p4
  Delay3 : Delay  DelayLength=1  InitialConditionSource=Input port  InitialCondition=0  ExternalReset=Rising  SampleTime=Ts
      settings: InputPortMap=u0,r5,p4
  From Workspace : FromWorkspace  VariableName=T_sim  SampleTime=Ts
  Unit Delay3 : UnitDelay  SampleTime=Ts
  YV2P : MATLAB Function  TreatAsAtomicUnit=on  SystemSampleTime=Ts
  Position : Outport
  wires:
  Velocities/1 -> YV2P/1(Velocity), Delay1/1
  HeadingAngles/1 -> Delay3/1, YV2P/3(Yaw)
  Delay2/1 -> YV2P/7(Lastpostion)
  Initial position/1 -> Delay2/3
  Iintial Velocities/1 -> Delay1/3
  Iintial HeadingAngles/1 -> Delay3/3
  From Workspace/1 -> YV2P/5(Tsim), Unit Delay3/1
  Delay1/1 -> YV2P/2(LastVelocity)
  Delay3/1 -> YV2P/4(LastYaw)
  Unit Delay3/1 -> YV2P/6(LastTsim)
  YV2P/1(Position) -> Delay2/1, Position/1
  select_overlap/1 -> Delay2/2, Delay1/2, Delay3/2

== system ISReferenceApplication/Subsystem_3/Subsystem/YV_update ==
  XY_sim : Inport
  Velocity_sim : Inport  Port=2
  Heading_sim : Inport  Port=3
  Constant : Constant  Value=Ts  SampleTime=Ts
  From Workspace1 : FromWorkspace  VariableName=T_sim  SampleTime=Ts
  From Workspace3 : FromWorkspace  VariableName=XY_Ref_Upd  SampleTime=Ts
  YV_update : MATLAB Function  TreatAsAtomicUnit=on  SystemSampleTime=Ts
  Velocity_updated : Outport
  Heading_updated : Outport  Port=2
  wires:
  YV_update/1(Velocity_updated) -> Velocity_updated/1
  From Workspace3/1 -> YV_update/1(XYplot_ref)
  YV_update/2(Heading_updated) -> Heading_updated/1
  From Workspace1/1 -> YV_update/6(Tsim)
  XY_sim/1 -> YV_update/2(XYplot_sim)
  Velocity_sim/1 -> YV_update/3(Velocity_sim)
  Heading_sim/1 -> YV_update/4(Heading_sim)
  Constant/1 -> YV_update/5(Ts)

== system ISReferenceApplication/Subsystem_4/Subsystem/MPC_of_simulator_4 ==
  Velocity_updated : Inport  SampleTime=Ts  LockScale=on
  Heading_updated : Inport  Port=2  SampleTime=Ts  LockScale=on
  select_MPC : Inport  Port=3  SampleTime=Ts  LockScale=on
  select_overlap : Inport  Port=4  SampleTime=Ts  LockScale=on
  U(k-1) : Inport  Port=5  SampleTime=Ts  LockScale=on
  Xhat : Inport  Port=6
  Clock : Clock
  Constant1 : Constant  Value=M  VectorParams1D=off  SampleTime=-1
  Constant2 : Constant  Value=Np  SampleTime=-1
  Constant3 : Constant  Value=JE_4  VectorParams1D=off  SampleTime=-1
  Constant4 : Constant  Value=Qc_4  VectorParams1D=off  SampleTime=-1
  Constant5 : Constant  Value=phi_4  VectorParams1D=off  SampleTime=-1
  Constant6 : Constant  Value=Tend  SampleTime=-1
  F_Middle : Gain  Gain=F_4  Multiplication=Matrix(K*u) (u vector)
  From Workspace6 : FromWorkspace  VariableName=Rs  SampleTime=Ts
  HQP : MATLAB Function  TreatAsAtomicUnit=on  SystemSampleTime=Ts
  Resettable Delay2 : Delay  DelayLength=1  InitialConditionSource=Input port  ExternalReset=Rising  SampleTime=Ts
      settings: InputPortMap=u0,r5,p4
  r(k+1) : Outport
  U : Outport  Port=2
  wires:
  HQP/2(U) -> Resettable Delay2/1, U/1
  Xhat/1 -> F_Middle/1
  Constant4/1 -> HQP/4(Qc)
  Constant5/1 -> HQP/2(phi)
  Constant3/1 -> HQP/1(JE)
  Constant2/1 -> HQP/6(Np)
  Constant1/1 -> HQP/5(M)
  Clock/1 -> HQP/10(Tsim)
  F_Middle/1 -> HQP/3(Fxh)
  From Workspace6/1 -> HQP/9(Rs)
  Heading_updated/1 -> HQP/7(Heading_updated)
  Velocity_updated/1 -> HQP/8(Velocity_updated)
  HQP/1(r) -> r(k+1)/1
  select_MPC/1 -> HQP/11(select_MPC)
  Resettable Delay2/1 -> HQP/13(U_delay)
  select_overlap/1 -> HQP/14(select_overlap), Resettable Delay2/2
  U(k-1)/1 -> Resettable Delay2/3
  Constant6/1 -> HQP/12(Tend)

== system ISReferenceApplication/Subsystem_4/Subsystem/VH2P ==
  Velocities : Inport
  HeadingAngles : Inport  Port=2
  Iintial Velocities : Inport  Port=3
  Iintial HeadingAngles : Inport  Port=4
  Initial position : Inport  Port=5
  select_overlap : Inport  Port=6
  Delay1 : Delay  DelayLength=1  InitialConditionSource=Input port  InitialCondition=0  ExternalReset=Rising  SampleTime=Ts
      settings: InputPortMap=u0,r5,p4
  Delay2 : Delay  DelayLength=1  InitialConditionSource=Input port  InitialCondition=0  ExternalReset=Rising  SampleTime=Ts
      settings: InputPortMap=u0,r5,p4
  Delay3 : Delay  DelayLength=1  InitialConditionSource=Input port  InitialCondition=0  ExternalReset=Rising  SampleTime=Ts
      settings: InputPortMap=u0,r5,p4
  From Workspace : FromWorkspace  VariableName=T_sim  SampleTime=Ts
  Unit Delay3 : UnitDelay  SampleTime=Ts
  YV2P : MATLAB Function  TreatAsAtomicUnit=on  SystemSampleTime=Ts
  Position : Outport
  wires:
  Velocities/1 -> YV2P/1(Velocity), Delay1/1
  HeadingAngles/1 -> Delay3/1, YV2P/3(Yaw)
  Delay2/1 -> YV2P/7(Lastpostion)
  Initial position/1 -> Delay2/3
  Iintial Velocities/1 -> Delay1/3
  Iintial HeadingAngles/1 -> Delay3/3
  From Workspace/1 -> YV2P/5(Tsim), Unit Delay3/1
  Delay1/1 -> YV2P/2(LastVelocity)
  Delay3/1 -> YV2P/4(LastYaw)
  Unit Delay3/1 -> YV2P/6(LastTsim)
  YV2P/1(Position) -> Delay2/1, Position/1
  select_overlap/1 -> Delay2/2, Delay1/2, Delay3/2

== system ISReferenceApplication/Subsystem_4/Subsystem/YV_update ==
  XY_sim : Inport
  Velocity_sim : Inport  Port=2
  Heading_sim : Inport  Port=3
  Constant : Constant  Value=Ts  SampleTime=Ts
  From Workspace1 : FromWorkspace  VariableName=T_sim  SampleTime=Ts
  From Workspace3 : FromWorkspace  VariableName=XY_Ref_Upd  SampleTime=Ts
  YV_update : MATLAB Function  TreatAsAtomicUnit=on  SystemSampleTime=Ts
  Velocity_updated : Outport
  Heading_updated : Outport  Port=2
  wires:
  YV_update/1(Velocity_updated) -> Velocity_updated/1
  From Workspace3/1 -> YV_update/1(XYplot_ref)
  YV_update/2(Heading_updated) -> Heading_updated/1
  From Workspace1/1 -> YV_update/6(Tsim)
  XY_sim/1 -> YV_update/2(XYplot_sim)
  Velocity_sim/1 -> YV_update/3(Velocity_sim)
  Heading_sim/1 -> YV_update/4(Heading_sim)
  Constant/1 -> YV_update/5(Ts)

== system ISReferenceApplication/Subsystem_5/Subsystem/MPC_of_simulator_5 ==
  Velocity_updated : Inport  SampleTime=Ts  LockScale=on
  Heading_updated : Inport  Port=2  SampleTime=Ts  LockScale=on
  select_MPC : Inport  Port=3  SampleTime=Ts  LockScale=on
  select_overlap : Inport  Port=4  SampleTime=Ts  LockScale=on
  U(k-1) : Inport  Port=5  SampleTime=Ts  LockScale=on
  Xhat : Inport  Port=6
  Clock : Clock
  Constant1 : Constant  Value=M  VectorParams1D=off  SampleTime=-1
  Constant2 : Constant  Value=Np  SampleTime=-1
  Constant3 : Constant  Value=JE_5  VectorParams1D=off  SampleTime=-1
  Constant4 : Constant  Value=Qc_5  VectorParams1D=off  SampleTime=-1
  Constant5 : Constant  Value=phi_5  VectorParams1D=off  SampleTime=-1
  Constant6 : Constant  Value=Tend  SampleTime=-1
  F_Middle : Gain  Gain=F_5  Multiplication=Matrix(K*u) (u vector)
  From Workspace6 : FromWorkspace  VariableName=Rs  SampleTime=Ts
  HQP : MATLAB Function  TreatAsAtomicUnit=on  SystemSampleTime=Ts
  Resettable Delay2 : Delay  DelayLength=1  InitialConditionSource=Input port  ExternalReset=Rising  SampleTime=Ts
      settings: InputPortMap=u0,r5,p4
  r(k+1) : Outport
  U : Outport  Port=2
  wires:
  HQP/2(U) -> Resettable Delay2/1, U/1
  Xhat/1 -> F_Middle/1
  Constant4/1 -> HQP/4(Qc)
  Constant5/1 -> HQP/2(phi)
  Constant3/1 -> HQP/1(JE)
  Constant2/1 -> HQP/6(Np)
  Constant1/1 -> HQP/5(M)
  Clock/1 -> HQP/10(Tsim)
  F_Middle/1 -> HQP/3(Fxh)
  From Workspace6/1 -> HQP/9(Rs)
  Heading_updated/1 -> HQP/7(Heading_updated)
  Velocity_updated/1 -> HQP/8(Velocity_updated)
  HQP/1(r) -> r(k+1)/1
  select_MPC/1 -> HQP/11(select_MPC)
  Resettable Delay2/1 -> HQP/13(U_delay)
  select_overlap/1 -> HQP/14(select_overlap), Resettable Delay2/2
  U(k-1)/1 -> Resettable Delay2/3
  Constant6/1 -> HQP/12(Tend)

== system ISReferenceApplication/Subsystem_5/Subsystem/VH2P ==
  Velocities : Inport
  HeadingAngles : Inport  Port=2
  Iintial Velocities : Inport  Port=3
  Iintial HeadingAngles : Inport  Port=4
  Initial position : Inport  Port=5
  select_overlap : Inport  Port=6
  Delay1 : Delay  DelayLength=1  InitialConditionSource=Input port  InitialCondition=0  ExternalReset=Rising  SampleTime=Ts
      settings: InputPortMap=u0,r5,p4
  Delay2 : Delay  DelayLength=1  InitialConditionSource=Input port  InitialCondition=0  ExternalReset=Rising  SampleTime=Ts
      settings: InputPortMap=u0,r5,p4
  Delay3 : Delay  DelayLength=1  InitialConditionSource=Input port  InitialCondition=0  ExternalReset=Rising  SampleTime=Ts
      settings: InputPortMap=u0,r5,p4
  From Workspace : FromWorkspace  VariableName=T_sim  SampleTime=Ts
  Unit Delay3 : UnitDelay  SampleTime=Ts
  YV2P : MATLAB Function  TreatAsAtomicUnit=on  SystemSampleTime=Ts
  Position : Outport
  wires:
  Velocities/1 -> YV2P/1(Velocity), Delay1/1
  HeadingAngles/1 -> Delay3/1, YV2P/3(Yaw)
  Delay2/1 -> YV2P/7(Lastpostion)
  Initial position/1 -> Delay2/3
  Iintial Velocities/1 -> Delay1/3
  Iintial HeadingAngles/1 -> Delay3/3
  From Workspace/1 -> YV2P/5(Tsim), Unit Delay3/1
  Delay1/1 -> YV2P/2(LastVelocity)
  Delay3/1 -> YV2P/4(LastYaw)
  Unit Delay3/1 -> YV2P/6(LastTsim)
  YV2P/1(Position) -> Delay2/1, Position/1
  select_overlap/1 -> Delay2/2, Delay1/2, Delay3/2

== system ISReferenceApplication/Subsystem_5/Subsystem/YV_update ==
  XY_sim : Inport
  Velocity_sim : Inport  Port=2
  Heading_sim : Inport  Port=3
  Constant : Constant  Value=Ts  SampleTime=Ts
  From Workspace1 : FromWorkspace  VariableName=T_sim  SampleTime=Ts
  From Workspace3 : FromWorkspace  VariableName=XY_Ref_Upd  SampleTime=Ts
  YV_update : MATLAB Function  TreatAsAtomicUnit=on  SystemSampleTime=Ts
  Velocity_updated : Outport
  Heading_updated : Outport  Port=2
  wires:
  YV_update/1(Velocity_updated) -> Velocity_updated/1
  From Workspace3/1 -> YV_update/1(XYplot_ref)
  YV_update/2(Heading_updated) -> Heading_updated/1
  From Workspace1/1 -> YV_update/6(Tsim)
  XY_sim/1 -> YV_update/2(XYplot_sim)
  Velocity_sim/1 -> YV_update/3(Velocity_sim)
  Heading_sim/1 -> YV_update/4(Heading_sim)
  Constant/1 -> YV_update/5(Ts)

== system ISReferenceApplication/Subsystem_6/Subsystem/MPC_of_simulator_6 ==
  Velocity_updated : Inport  SampleTime=Ts  LockScale=on
  Heading_updated : Inport  Port=2  SampleTime=Ts  LockScale=on
  select_MPC : Inport  Port=3  SampleTime=Ts  LockScale=on
  select_overlap : Inport  Port=4  SampleTime=Ts  LockScale=on
  U(k-1) : Inport  Port=5  SampleTime=Ts  LockScale=on
  Xhat : Inport  Port=6
  Clock : Clock
  Constant1 : Constant  Value=M  VectorParams1D=off  SampleTime=-1
  Constant2 : Constant  Value=Np  SampleTime=-1
  Constant3 : Constant  Value=JE_6  VectorParams1D=off  SampleTime=-1
  Constant4 : Constant  Value=Qc_6  VectorParams1D=off  SampleTime=-1
  Constant5 : Constant  Value=phi_6  VectorParams1D=off  SampleTime=-1
  Constant6 : Constant  Value=Tend  SampleTime=-1
  F_Middle : Gain  Gain=F_6  Multiplication=Matrix(K*u) (u vector)
  From Workspace6 : FromWorkspace  VariableName=Rs  SampleTime=Ts
  HQP : MATLAB Function  TreatAsAtomicUnit=on  SystemSampleTime=Ts
  Resettable Delay2 : Delay  DelayLength=1  InitialConditionSource=Input port  ExternalReset=Rising  SampleTime=Ts
      settings: InputPortMap=u0,r5,p4
  r(k+1) : Outport
  U : Outport  Port=2
  wires:
  HQP/2(U) -> Resettable Delay2/1, U/1
  Xhat/1 -> F_Middle/1
  Constant4/1 -> HQP/4(Qc)
  Constant5/1 -> HQP/2(phi)
  Constant3/1 -> HQP/1(JE)
  Constant2/1 -> HQP/6(Np)
  Constant1/1 -> HQP/5(M)
  Clock/1 -> HQP/10(Tsim)
  F_Middle/1 -> HQP/3(Fxh)
  From Workspace6/1 -> HQP/9(Rs)
  Heading_updated/1 -> HQP/7(Heading_updated)
  Velocity_updated/1 -> HQP/8(Velocity_updated)
  HQP/1(r) -> r(k+1)/1
  select_MPC/1 -> HQP/11(select_MPC)
  Resettable Delay2/1 -> HQP/13(U_delay)
  select_overlap/1 -> HQP/14(select_overlap), Resettable Delay2/2
  U(k-1)/1 -> Resettable Delay2/3
  Constant6/1 -> HQP/12(Tend)

== system ISReferenceApplication/Subsystem_6/Subsystem/VH2P ==
  Velocities : Inport
  HeadingAngles : Inport  Port=2
  Iintial Velocities : Inport  Port=3
  Iintial HeadingAngles : Inport  Port=4
  Initial position : Inport  Port=5
  select_overlap : Inport  Port=6
  Delay1 : Delay  DelayLength=1  InitialConditionSource=Input port  InitialCondition=0  ExternalReset=Rising  SampleTime=Ts
      settings: InputPortMap=u0,r5,p4
  Delay2 : Delay  DelayLength=1  InitialConditionSource=Input port  InitialCondition=0  ExternalReset=Rising  SampleTime=Ts
      settings: InputPortMap=u0,r5,p4
  Delay3 : Delay  DelayLength=1  InitialConditionSource=Input port  InitialCondition=0  ExternalReset=Rising  SampleTime=Ts
      settings: InputPortMap=u0,r5,p4
  From Workspace : FromWorkspace  VariableName=T_sim  SampleTime=Ts
  Unit Delay3 : UnitDelay  SampleTime=Ts
  YV2P : MATLAB Function  TreatAsAtomicUnit=on  SystemSampleTime=Ts
  Position : Outport
  wires:
  Velocities/1 -> YV2P/1(Velocity), Delay1/1
  HeadingAngles/1 -> Delay3/1, YV2P/3(Yaw)
  Delay2/1 -> YV2P/7(Lastpostion)
  Initial position/1 -> Delay2/3
  Iintial Velocities/1 -> Delay1/3
  Iintial HeadingAngles/1 -> Delay3/3
  From Workspace/1 -> YV2P/5(Tsim), Unit Delay3/1
  Delay1/1 -> YV2P/2(LastVelocity)
  Delay3/1 -> YV2P/4(LastYaw)
  Unit Delay3/1 -> YV2P/6(LastTsim)
  YV2P/1(Position) -> Delay2/1, Position/1
  select_overlap/1 -> Delay2/2, Delay1/2, Delay3/2

== system ISReferenceApplication/Subsystem_6/Subsystem/YV_update ==
  XY_sim : Inport
  Velocity_sim : Inport  Port=2
  Heading_sim : Inport  Port=3
  Constant : Constant  Value=Ts  SampleTime=Ts
  From Workspace1 : FromWorkspace  VariableName=T_sim  SampleTime=Ts
  From Workspace3 : FromWorkspace  VariableName=XY_Ref_Upd  SampleTime=Ts
  YV_update : MATLAB Function  TreatAsAtomicUnit=on  SystemSampleTime=Ts
  Velocity_updated : Outport
  Heading_updated : Outport  Port=2
  wires:
  YV_update/1(Velocity_updated) -> Velocity_updated/1
  From Workspace3/1 -> YV_update/1(XYplot_ref)
  YV_update/2(Heading_updated) -> Heading_updated/1
  From Workspace1/1 -> YV_update/6(Tsim)
  XY_sim/1 -> YV_update/2(XYplot_sim)
  Velocity_sim/1 -> YV_update/3(Velocity_sim)
  Heading_sim/1 -> YV_update/4(Heading_sim)
  Constant/1 -> YV_update/5(Ts)

== system ISReferenceApplication/Subsystem_7/Subsystem/MPC_of_simulator_7 ==
  Velocity_updated : Inport  SampleTime=Ts  LockScale=on
  Heading_updated : Inport  Port=2  SampleTime=Ts  LockScale=on
  select_MPC : Inport  Port=3  SampleTime=Ts  LockScale=on
  select_overlap : Inport  Port=4  SampleTime=Ts  LockScale=on
  U(k-1) : Inport  Port=5  SampleTime=Ts  LockScale=on
  Xhat : Inport  Port=6
  Clock : Clock
  Constant1 : Constant  Value=M  VectorParams1D=off  SampleTime=-1
  Constant2 : Constant  Value=Np  SampleTime=-1
  Constant3 : Constant  Value=JE_7  VectorParams1D=off  SampleTime=-1
  Constant4 : Constant  Value=Qc_7  VectorParams1D=off  SampleTime=-1
  Constant5 : Constant  Value=phi_7  VectorParams1D=off  SampleTime=-1
  Constant6 : Constant  Value=Tend  SampleTime=-1
  F_Middle : Gain  Gain=F_7  Multiplication=Matrix(K*u) (u vector)
  From Workspace6 : FromWorkspace  VariableName=Rs  SampleTime=Ts
  HQP : MATLAB Function  TreatAsAtomicUnit=on  SystemSampleTime=Ts
  Resettable Delay2 : Delay  DelayLength=1  InitialConditionSource=Input port  ExternalReset=Rising  SampleTime=Ts
      settings: InputPortMap=u0,r5,p4
  r(k+1) : Outport
  U : Outport  Port=2
  wires:
  HQP/2(U) -> Resettable Delay2/1, U/1
  Xhat/1 -> F_Middle/1
  Constant4/1 -> HQP/4(Qc)
  Constant5/1 -> HQP/2(phi)
  Constant3/1 -> HQP/1(JE)
  Constant2/1 -> HQP/6(Np)
  Constant1/1 -> HQP/5(M)
  Clock/1 -> HQP/10(Tsim)
  F_Middle/1 -> HQP/3(Fxh)
  From Workspace6/1 -> HQP/9(Rs)
  Heading_updated/1 -> HQP/7(Heading_updated)
  Velocity_updated/1 -> HQP/8(Velocity_updated)
  HQP/1(r) -> r(k+1)/1
  select_MPC/1 -> HQP/11(select_MPC)
  Resettable Delay2/1 -> HQP/13(U_delay)
  select_overlap/1 -> HQP/14(select_overlap), Resettable Delay2/2
  U(k-1)/1 -> Resettable Delay2/3
  Constant6/1 -> HQP/12(Tend)
